simulink model "satnodemodel"  (Simulink 7.0)
settings: Solver=ode45  StartTime=0.0  StopTime=10.0  RelTol=1e-6
undefined symbols (not defined in the file or in its folder): x, xdot
settings Model: Creator=abbas  LastModifiedBy=abbas
settings OptimizationCC: InlineInvariantSignals=on
settings DebuggingCC: SaveWithParameterizedLinksMsg=none  SignalResolutionControl=TryResolveAllWithWarning  SolverPrmCheckMsg=none  MultiTaskDSMMsg=warning  MultiTaskCondExecSysMsg=none  StrictBusMsg=None
settings RTWCC: IncludeERTFirstTime=on
settings GRTTargetCC: TargetFcnLib=ansi_tfl_tmw.mat

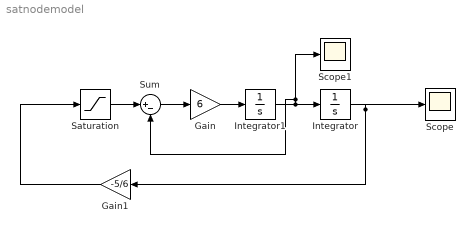
== system satnodemodel ==
  Gain : Gain  Gain=6  ParameterDataType=sfix(16)  ParameterScaling=2^0  OutDataType=sfix(16)  OutScaling=2^0
  Gain1 : Gain  Orientation=left  Gain=-5/6  ParameterDataType=sfix(16)  ParameterScaling=2^0  OutDataType=sfix(16)  OutScaling=2^0
  Integrator : Integrator  InitialCondition=x
  Integrator1 : Integrator  InitialCondition=xdot
  Saturation : Saturate  UpperLimit=.5  LowerLimit=-.5
  Scope : Scope
      settings: SaveName=xsat  DataFormat=Array
  Scope1 : Scope
      settings: SaveName=xdotsat  DataFormat=Array
  Sum : Sum  Inputs=|+-  OutDataType=sfix(16)  OutScaling=2^0
  wires:
  Integrator1/1 -> Integrator/1, Scope1/1, Sum/2
  Integrator/1 -> Gain1/1, Scope/1
  Gain1/1 -> Saturation/1
  Saturation/1 -> Sum/1
  Sum/1 -> Gain/1
  Gain/1 -> Integrator1/1
